simulink model "gm_Encoder_Zynq_vnl"  (R2018a)
settings: Solver=ode3  StartTime=0.0  StopTime=SimulationsDauer  RelTol=1e-3  EnableMultiTasking=on
undefined symbols (not defined in the file or in its folder): DiscIntNeverNeededParam, f_ISR, IncPerTurn, n_max, OverSamplingFactor, OverSamplingFactorInverse, Periode, Phase_Delay_A, Phase_Delay_B, PolePair, T_mech, TestDrehzahl_rpm
libraries: simulink x18, hdlsllib x2, dspsigops x2, dspswit3 x2, powerlib_meascontrol x2, hdlmdlgenlib x1, simulink_extras x1, powerlib x1
(part 2 of 3)

== system gm_Encoder_Zynq_vnl/Compare/Assert_edge ==
  cosim : Inport
  dut : Inport  Port=2
  AssertEq : Assertion  StopWhenAssertionFail=off
  Compare To Zero : simulink/Logic and Bit Operations/Compare To Zero  relop===  OutDataTypeStr=boolean
  Constant1 : Constant  Value=0  OutDataTypeStr=Inherit: Inherit via back propagation  SampleTime=-1
  Counter : simulink/Sources/Counter Free-Running  NumBits=32  tsamp=-1
  IgnoreCycles : Constant  Value=11  OutDataTypeStr=Inherit: Inherit via back propagation  SampleTime=-1
  Relational Operator : RelationalOperator  Operator=<  OutDataTypeStr=boolean  RndMeth=Nearest
  Relational Operator1 : RelationalOperator  Operator===  OutDataTypeStr=boolean  RndMeth=Nearest
  Switch : Switch  Criteria=u2 ~= 0
  Switch1 : Switch  Criteria=u2 ~= 0
  compare: edge : Scope  NumInputPorts=3
  wires:
  Compare To Zero/1 -> compare: edge/3
  Relational Operator1/1 -> Compare To Zero/1, AssertEq/1  "err"
  Switch1/1 -> compare: edge/1, Relational Operator1/1
  Switch/1 -> compare: edge/2, Relational Operator1/2
  Constant1/1 -> Switch/1, Switch1/1
  Relational Operator/1 -> Switch/2, Switch1/2
  cosim/1 -> Switch1/3  "cosim"
  dut/1 -> Switch/3  "dut ref"
  Counter/1 -> Relational Operator/1
  IgnoreCycles/1 -> Relational Operator/2

== system gm_Encoder_Zynq_vnl/Compare/Assert_omega ==
  cosim : Inport
  dut : Inport  Port=2
  AssertEq : Assertion  StopWhenAssertionFail=off
  Compare To Zero : simulink/Logic and Bit Operations/Compare To Zero  relop===  OutDataTypeStr=boolean
  Constant1 : Constant  Value=0  OutDataTypeStr=Inherit: Inherit via back propagation  SampleTime=-1
  Counter : simulink/Sources/Counter Free-Running  NumBits=32  tsamp=-1
  IgnoreCycles : Constant  Value=11  OutDataTypeStr=Inherit: Inherit via back propagation  SampleTime=-1
  Relational Operator : RelationalOperator  Operator=<  OutDataTypeStr=boolean  RndMeth=Nearest
  Relational Operator1 : RelationalOperator  Operator===  OutDataTypeStr=boolean  RndMeth=Nearest
  Switch : Switch  Criteria=u2 ~= 0
  Switch1 : Switch  Criteria=u2 ~= 0
  compare: omega : Scope  NumInputPorts=3
  wires:
  Compare To Zero/1 -> compare: omega/3
  Relational Operator1/1 -> Compare To Zero/1, AssertEq/1  "err"
  Switch1/1 -> compare: omega/1, Relational Operator1/1
  Switch/1 -> compare: omega/2, Relational Operator1/2
  Constant1/1 -> Switch/1, Switch1/1
  Relational Operator/1 -> Switch/2, Switch1/2
  cosim/1 -> Switch1/3  "cosim"
  dut/1 -> Switch/3  "dut ref"
  Counter/1 -> Relational Operator/1
  IgnoreCycles/1 -> Relational Operator/2

== system gm_Encoder_Zynq_vnl/Compare/Assert_omega_AXI4 ==
  cosim : Inport
  dut : Inport  Port=2
  AssertEq : Assertion  StopWhenAssertionFail=off
  Compare To Zero : simulink/Logic and Bit Operations/Compare To Zero  relop===  OutDataTypeStr=boolean
  Constant1 : Constant  Value=0  OutDataTypeStr=Inherit: Inherit via back propagation  SampleTime=-1
  Counter : simulink/Sources/Counter Free-Running  NumBits=32  tsamp=-1
  IgnoreCycles : Constant  Value=11  OutDataTypeStr=Inherit: Inherit via back propagation  SampleTime=-1
  Relational Operator : RelationalOperator  Operator=<  OutDataTypeStr=boolean  RndMeth=Nearest
  Relational Operator1 : RelationalOperator  Operator===  OutDataTypeStr=boolean  RndMeth=Nearest
  Switch : Switch  Criteria=u2 ~= 0
  Switch1 : Switch  Criteria=u2 ~= 0
  compare: omega_AXI4 : Scope  NumInputPorts=3
  wires:
  Compare To Zero/1 -> compare: omega_AXI4/3
  Relational Operator1/1 -> Compare To Zero/1, AssertEq/1  "err"
  Switch1/1 -> compare: omega_AXI4/1, Relational Operator1/1
  Switch/1 -> compare: omega_AXI4/2, Relational Operator1/2
  Constant1/1 -> Switch/1, Switch1/1
  Relational Operator/1 -> Switch/2, Switch1/2
  cosim/1 -> Switch1/3  "cosim"
  dut/1 -> Switch/3  "dut ref"
  Counter/1 -> Relational Operator/1
  IgnoreCycles/1 -> Relational Operator/2

== system gm_Encoder_Zynq_vnl/Compare/Assert_theta_el ==
  cosim : Inport
  dut : Inport  Port=2
  AssertEq : Assertion  StopWhenAssertionFail=off
  Compare To Zero : simulink/Logic and Bit Operations/Compare To Zero  relop===  OutDataTypeStr=boolean
  Constant1 : Constant  Value=0  OutDataTypeStr=Inherit: Inherit via back propagation  SampleTime=-1
  Counter : simulink/Sources/Counter Free-Running  NumBits=32  tsamp=-1
  IgnoreCycles : Constant  Value=11  OutDataTypeStr=Inherit: Inherit via back propagation  SampleTime=-1
  Relational Operator : RelationalOperator  Operator=<  OutDataTypeStr=boolean  RndMeth=Nearest
  Relational Operator1 : RelationalOperator  Operator===  OutDataTypeStr=boolean  RndMeth=Nearest
  Switch : Switch  Criteria=u2 ~= 0
  Switch1 : Switch  Criteria=u2 ~= 0
  compare: theta_el : Scope  NumInputPorts=3
  wires:
  Compare To Zero/1 -> compare: theta_el/3
  Relational Operator1/1 -> Compare To Zero/1, AssertEq/1  "err"
  Switch1/1 -> compare: theta_el/1, Relational Operator1/1
  Switch/1 -> compare: theta_el/2, Relational Operator1/2
  Constant1/1 -> Switch/1, Switch1/1
  Relational Operator/1 -> Switch/2, Switch1/2
  cosim/1 -> Switch1/3  "cosim"
  dut/1 -> Switch/3  "dut ref"
  Counter/1 -> Relational Operator/1
  IgnoreCycles/1 -> Relational Operator/2

== system gm_Encoder_Zynq_vnl/Compare/Assert_theta_el_AXI4 ==
  cosim : Inport
  dut : Inport  Port=2
  AssertEq : Assertion  StopWhenAssertionFail=off
  Compare To Zero : simulink/Logic and Bit Operations/Compare To Zero  relop===  OutDataTypeStr=boolean
  Constant1 : Constant  Value=0  OutDataTypeStr=Inherit: Inherit via back propagation  SampleTime=-1
  Counter : simulink/Sources/Counter Free-Running  NumBits=32  tsamp=-1
  IgnoreCycles : Constant  Value=11  OutDataTypeStr=Inherit: Inherit via back propagation  SampleTime=-1
  Relational Operator : RelationalOperator  Operator=<  OutDataTypeStr=boolean  RndMeth=Nearest
  Relational Operator1 : RelationalOperator  Operator===  OutDataTypeStr=boolean  RndMeth=Nearest
  Switch : Switch  Criteria=u2 ~= 0
  Switch1 : Switch  Criteria=u2 ~= 0
  compare: theta_el_AXI4 : Scope  NumInputPorts=3
  wires:
  Compare To Zero/1 -> compare: theta_el_AXI4/3
  Relational Operator1/1 -> Compare To Zero/1, AssertEq/1  "err"
  Switch1/1 -> compare: theta_el_AXI4/1, Relational Operator1/1
  Switch/1 -> compare: theta_el_AXI4/2, Relational Operator1/2
  Constant1/1 -> Switch/1, Switch1/1
  Relational Operator/1 -> Switch/2, Switch1/2
  cosim/1 -> Switch1/3  "cosim"
  dut/1 -> Switch/3  "dut ref"
  Counter/1 -> Relational Operator/1
  IgnoreCycles/1 -> Relational Operator/2

== system gm_Encoder_Zynq_vnl/Compare/Assert_theta_mech_AXI4 ==
  cosim : Inport
  dut : Inport  Port=2
  AssertEq : Assertion  StopWhenAssertionFail=off
  Compare To Zero : simulink/Logic and Bit Operations/Compare To Zero  relop===  OutDataTypeStr=boolean
  Constant1 : Constant  Value=0  OutDataTypeStr=Inherit: Inherit via back propagation  SampleTime=-1
  Counter : simulink/Sources/Counter Free-Running  NumBits=32  tsamp=-1
  IgnoreCycles : Constant  Value=11  OutDataTypeStr=Inherit: Inherit via back propagation  SampleTime=-1
  Relational Operator : RelationalOperator  Operator=<  OutDataTypeStr=boolean  RndMeth=Nearest
  Relational Operator1 : RelationalOperator  Operator===  OutDataTypeStr=boolean  RndMeth=Nearest
  Switch : Switch  Criteria=u2 ~= 0
  Switch1 : Switch  Criteria=u2 ~= 0
  compare: theta_mech_AXI4 : Scope  NumInputPorts=3
  wires:
  Compare To Zero/1 -> compare: theta_mech_AXI4/3
  Relational Operator1/1 -> Compare To Zero/1, AssertEq/1  "err"
  Switch1/1 -> compare: theta_mech_AXI4/1, Relational Operator1/1
  Switch/1 -> compare: theta_mech_AXI4/2, Relational Operator1/2
  Constant1/1 -> Switch/1, Switch1/1
  Relational Operator/1 -> Switch/2, Switch1/2
  cosim/1 -> Switch1/3  "cosim"
  dut/1 -> Switch/3  "dut ref"
  Counter/1 -> Relational Operator/1
  IgnoreCycles/1 -> Relational Operator/2

== system gm_Encoder_Zynq_vnl/Compare/CleanupScopes ==

== system gm_Encoder_Zynq_vnl/Compare/Enable ==

== system gm_Encoder_Zynq_vnl/IncreEncoder_V16/Check_Direction ==
  A : Inport
  B : Inport  Port=2
  Add : Sum  Inputs=+-  AccumDataTypeStr=fixdt(1,4,0)  OutDataTypeStr=fixdt(1,4,0)
  Add1 : Sum  Inputs=+-  AccumDataTypeStr=fixdt(1,4,0)  OutDataTypeStr=fixdt(1,4,0)
  Add2 : Sum  AccumDataTypeStr=fixdt(1,4,0)  OutDataTypeStr=fixdt(1,4,0)
  Change : Sum  AccumDataTypeStr=fixdt(1,4,0)  OutDataTypeStr=fixdt(1,4,0)
  Change1 : Delay  DelayLength=1
  Save_Direction : Switch  Criteria=u2 ~= 0  Threshold=0.1  OutDataTypeStr=Inherit: Inherit via back propagation
  Scope6 : Scope  NumInputPorts=4
  T_count_switch : Switch  Threshold=1  OutDataTypeStr=Inherit: Inherit via back propagation
  TrnLeft : Sum  Inputs=+-  AccumDataTypeStr=fixdt(1,4,0)  OutDataTypeStr=fixdt(1,4,0)
  TrnRight : Sum  Inputs=+-  AccumDataTypeStr=fixdt(1,4,0)  OutDataTypeStr=fixdt(1,4,0)
  TurnLeft : Constant  Value=-1  OutDataTypeStr=fixdt(1,4,0)  SampleTime=-1
  TurnRight : Constant  OutDataTypeStr=fixdt(1,4,0)  SampleTime=-1
  count_old : Delay  DelayLength=1
  count_old1 : Delay  DelayLength=1
  count_old2 : Delay  DelayLength=1
  count_old_switch : Switch  Criteria=u2 ~= 0  OutDataTypeStr=Inherit: Inherit via back propagation
  count_old_switch1 : Switch  Criteria=u2 ~= 0  OutDataTypeStr=Inherit: Inherit via back propagation
  new_value : Delay  DelayLength=1
  nothing : Constant  Value=0  OutDataTypeStr=fixdt(1,4,0)  SampleTime=-1
  nothing1 : Constant  Value=0  OutDataTypeStr=fixdt(1,4,0)  SampleTime=-1
  speed_old_switch : Switch  Threshold=1  OutDataTypeStr=Inherit: Inherit via back propagation
  Dir : Outport
  wires:
  A/1 -> TrnLeft/2, Add/1, count_old_switch/1
  count_old_switch/1 -> count_old/1
  count_old/1 -> count_old_switch/3, Add/2
  TurnRight/1 -> T_count_switch/1
  Add/1 -> TrnRight/1, count_old_switch/2
  T_count_switch/1 -> Change/1, Add2/1
  Save_Direction/1 -> count_old2/1
  B/1 -> TrnRight/2, Add1/1, count_old_switch1/1
  count_old_switch1/1 -> count_old1/1
  count_old1/1 -> count_old_switch1/3, Add1/2
  Add1/1 -> TrnLeft/1, count_old_switch1/2
  TrnRight/1 -> Scope6/1, T_count_switch/2
  new_value/1 -> Save_Direction/1
  TrnLeft/1 -> speed_old_switch/2, Scope6/2
  TurnLeft/1 -> speed_old_switch/1
  nothing/1 -> speed_old_switch/3
  nothing1/1 -> T_count_switch/3
  speed_old_switch/1 -> Change/2, Add2/2
  Add2/1 -> Scope6/4, new_value/1
  Change/1 -> Change1/1
  Change1/1 -> Scope6/3, Save_Direction/2
  count_old2/1 -> Save_Direction/3, Dir/1

== system gm_Encoder_Zynq_vnl/IncreEncoder_V16/Counter_speed ==
  note: 1 for one cycle if edge recognized
  note: Check if count is to small
  note: Check if count is to big
  note: Reset
  note: Count
  Enable_ctr : Inport
  Reset : Inport  Port=2
  IncsPerTurn : Inport  Port=3
  Add1 : Sum  AccumDataTypeStr=int16  OutDataTypeStr=uint16
  Constant1 : Constant  Value=0  OutDataTypeStr=uint16  SampleTime=-1
  Constant2 : Constant  OutDataTypeStr=int8  SampleTime=-1
  Constant3 : Constant  Value=0  OutDataTypeStr=int8  SampleTime=-1
  Constant4 : Constant  Value=10  OutDataTypeStr=uint16  SampleTime=-1
  Detec_edge : Sum  Inputs=+-  AccumDataTypeStr=int8  OutDataTypeStr=int8
  Relational Operator : RelationalOperator  OutDataTypeStr=boolean  RndMeth=Nearest
  Reset_flag : Sum  Inputs=+-  AccumDataTypeStr=uint8  OutDataTypeStr=uint8
  Reset_when_overflow : Sum
  Resett_switch1 : Switch  Criteria=u2 ~= 0
  Resett_switch2 : Switch  Criteria=u2 ~= 0
  reset_old{,1..3} (4 alike) : Delay  DelayLength=1
  reset_old_switch : Switch  Criteria=u2 ~= 0
  reset_old_switch1 : Switch  Criteria=u2 ~= 0
  speed_old_switch1 : Switch  Threshold=1
  count : Outport
  wires:
  Reset/1 -> Reset_flag/1, reset_old_switch/1
  reset_old_switch/1 -> reset_old/1
  reset_old/1 -> reset_old_switch/3, Reset_flag/2
  Reset_flag/1 -> reset_old_switch/2, Resett_switch2/2
  Enable_ctr/1 -> Detec_edge/1, reset_old_switch1/1
  reset_old_switch1/1 -> reset_old1/1
  reset_old1/1 -> reset_old_switch1/3, Detec_edge/2
  Detec_edge/1 -> speed_old_switch1/2, reset_old_switch1/2  "1 for one cycle if edge recognized"
  Add1/1 -> Resett_switch2/3
  reset_old2/1 -> Relational Operator/1, Add1/2, count/1
  speed_old_switch1/1 -> Add1/1
  Constant3/1 -> speed_old_switch1/3
  Constant2/1 -> speed_old_switch1/1
  Constant4/1 -> Reset_when_overflow/1
  Reset_when_overflow/1 -> reset_old3/1
  Resett_switch1/1 -> reset_old2/1
  Relational Operator/1 -> Resett_switch1/2
  Constant1/1 -> Resett_switch2/1, Resett_switch1/1
  IncsPerTurn/1 -> Reset_when_overflow/2
  Resett_switch2/1 -> Resett_switch1/3
  reset_old3/1 -> Relational Operator/2

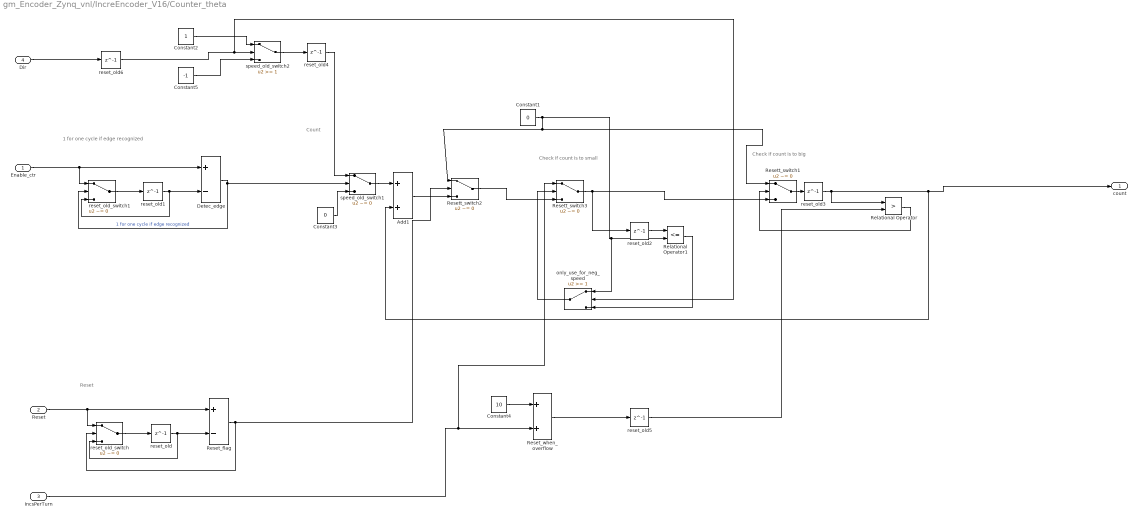
== system gm_Encoder_Zynq_vnl/IncreEncoder_V16/Counter_theta ==
  note: 1 for one cycle if edge recognized
  note: Reset
  note: Count
  note: Check if count is to big
  note: Check if count is to small
  Enable_ctr : Inport
  Reset : Inport  Port=2
  IncsPerTurn : Inport  Port=3
  Dir : Inport  Port=4
  Add1 : Sum  AccumDataTypeStr=int16  OutDataTypeStr=int16
  Constant1 : Constant  Value=0  OutDataTypeStr=int16  SampleTime=-1
  Constant2 : Constant  OutDataTypeStr=int16  SampleTime=-1
  Constant3 : Constant  Value=0  OutDataTypeStr=int16  SampleTime=-1
  Constant4 : Constant  Value=10  OutDataTypeStr=int16  SampleTime=-1
  Constant5 : Constant  Value=-1  OutDataTypeStr=int16  SampleTime=-1
  Detec_edge : Sum  Inputs=+-  AccumDataTypeStr=int8  OutDataTypeStr=int8
  Relational Operator : RelationalOperator  Operator=>  OutDataTypeStr=boolean  RndMeth=Nearest
  Relational Operator1 : RelationalOperator  Operator=<=  OutDataTypeStr=boolean  RndMeth=Nearest
  Reset_flag : Sum  Inputs=+-  AccumDataTypeStr=uint8  OutDataTypeStr=uint8
  Reset_when_overflow : Sum  OutDataTypeStr=int16
  Resett_switch1 : Switch  Criteria=u2 ~= 0  OutDataTypeStr=int16
  Resett_switch2 : Switch  Criteria=u2 ~= 0  OutDataTypeStr=int16
  Resett_switch3 : Switch  Criteria=u2 ~= 0  OutDataTypeStr=int16
  only_use_for_neg_speed : Switch  Threshold=1
  reset_old{,1..6} (7 alike) : Delay  DelayLength=1
  reset_old_switch : Switch  Criteria=u2 ~= 0
  reset_old_switch1 : Switch  Criteria=u2 ~= 0
  speed_old_switch1 : Switch  Criteria=u2 ~= 0
  speed_old_switch2 : Switch  Threshold=1
  count : Outport
  wires:
  Reset/1 -> Reset_flag/1, reset_old_switch/1
  reset_old_switch/1 -> reset_old/1
  reset_old/1 -> reset_old_switch/3, Reset_flag/2
  Reset_flag/1 -> reset_old_switch/2, Resett_switch2/2
  Enable_ctr/1 -> Detec_edge/1, reset_old_switch1/1
  reset_old_switch1/1 -> reset_old1/1
  reset_old1/1 -> reset_old_switch1/3, Detec_edge/2
  Detec_edge/1 -> speed_old_switch1/2, reset_old_switch1/2  "1 for one cycle if edge recognized"
  Add1/1 -> Resett_switch2/3
  speed_old_switch1/1 -> Add1/1
  Constant3/1 -> speed_old_switch1/3
  Constant2/1 -> speed_old_switch2/1
  Constant4/1 -> Reset_when_overflow/1
  Reset_when_overflow/1 -> reset_old5/1
  IncsPerTurn/1 -> Resett_switch3/1, Reset_when_overflow/2
  Dir/1 -> reset_old6/1
  Constant5/1 -> speed_old_switch2/3
  speed_old_switch2/1 -> reset_old4/1
  reset_old3/1 -> Add1/2, count/1, Relational Operator/1
  Resett_switch1/1 -> reset_old3/1
  Relational Operator/1 -> Resett_switch1/2
  Constant1/1 -> Resett_switch2/1, Resett_switch1/1, only_use_for_neg_speed/1, Relational Operator1/2
  Resett_switch3/1 -> reset_old2/1, Resett_switch1/3
  Resett_switch2/1 -> Resett_switch3/3
  reset_old2/1 -> Relational Operator1/1
  Relational Operator1/1 -> only_use_for_neg_speed/3
  only_use_for_neg_speed/1 -> Resett_switch3/2
  reset_old4/1 -> speed_old_switch1/1
  reset_old5/1 -> Relational Operator/2
  reset_old6/1 -> only_use_for_neg_speed/2, speed_old_switch2/2

== system gm_Encoder_Zynq_vnl/IncreEncoder_V16/Counter_theta_ele ==
  note: 1 for one cycle if edge recognized
  note: Reset
  note: Count
  note: Check if count is to big
  note: Check if count is to small
  Enable_ctr : Inport
  Reset : Inport  Port=2
  IncsPerTurn : Inport  Port=3
  Dir : Inport  Port=4
  Add1 : Sum  AccumDataTypeStr=int16  OutDataTypeStr=int16
  Constant1 : Constant  Value=0  OutDataTypeStr=int16  SampleTime=-1
  Constant2 : Constant  OutDataTypeStr=int16  SampleTime=-1
  Constant3 : Constant  Value=0  OutDataTypeStr=int16  SampleTime=-1
  Constant5 : Constant  Value=-1  OutDataTypeStr=int16  SampleTime=-1
  Detec_edge : Sum  Inputs=+-  AccumDataTypeStr=int8  OutDataTypeStr=int8
  Relational Operator : RelationalOperator  Operator=>  OutDataTypeStr=boolean  RndMeth=Nearest
  Relational Operator1 : RelationalOperator  Operator=<=  OutDataTypeStr=boolean  RndMeth=Nearest
  Reset_flag : Sum  Inputs=+-  AccumDataTypeStr=uint8  OutDataTypeStr=uint8
  Resett_switch1 : Switch  Criteria=u2 ~= 0  OutDataTypeStr=int16
  Resett_switch2 : Switch  Criteria=u2 ~= 0  OutDataTypeStr=int16
  Resett_switch3 : Switch  Criteria=u2 ~= 0  OutDataTypeStr=int16
  only_use_for_neg_speed : Switch  Threshold=1
  reset_old{,1..5} (6 alike) : Delay  DelayLength=1
  reset_old_switch : Switch  Criteria=u2 ~= 0
  reset_old_switch1 : Switch  Criteria=u2 ~= 0
  speed_old_switch1 : Switch  Criteria=u2 ~= 0
  speed_old_switch2 : Switch  Threshold=1
  count : Outport
  wires:
  Reset/1 -> Reset_flag/1, reset_old_switch/1
  reset_old_switch/1 -> reset_old/1
  reset_old/1 -> reset_old_switch/3, Reset_flag/2
  Reset_flag/1 -> reset_old_switch/2, Resett_switch2/2
  Enable_ctr/1 -> Detec_edge/1, reset_old_switch1/1
  reset_old_switch1/1 -> reset_old1/1
  reset_old1/1 -> reset_old_switch1/3, Detec_edge/2
  Detec_edge/1 -> speed_old_switch1/2, reset_old_switch1/2  "1 for one cycle if edge recognized"
  Add1/1 -> Resett_switch2/3
  speed_old_switch1/1 -> Add1/1
  Constant3/1 -> speed_old_switch1/3
  Constant2/1 -> speed_old_switch2/1
  IncsPerTurn/1 -> Resett_switch3/1, Relational Operator/2
  Dir/1 -> reset_old5/1
  Constant5/1 -> speed_old_switch2/3
  speed_old_switch2/1 -> reset_old4/1
  reset_old3/1 -> Add1/2, count/1, Relational Operator/1
  Resett_switch1/1 -> reset_old3/1
  Relational Operator/1 -> Resett_switch1/2
  Constant1/1 -> Resett_switch2/1, only_use_for_neg_speed/1, Relational Operator1/2, Resett_switch1/1
  Resett_switch3/1 -> reset_old2/1, Resett_switch1/3
  Resett_switch2/1 -> Resett_switch3/3
  reset_old2/1 -> Relational Operator1/1
  Relational Operator1/1 -> only_use_for_neg_speed/3
  only_use_for_neg_speed/1 -> Resett_switch3/2
  reset_old4/1 -> speed_old_switch1/1
  reset_old5/1 -> speed_old_switch2/2, only_use_for_neg_speed/2

== system gm_Encoder_Zynq_vnl/IncreEncoder_V16/n_aus_theta ==
  count : Inport
  IncsPerTurn : Inport  Port=2
  T : Inport  Port=3
  Add : Sum  Inputs=+-
  Add1 : Sum
  Constant : Constant  Value=0  OutDataTypeStr=fixdt(0,30,24)  SampleTime=-1
  Constant1 : Constant  Value=0  OutDataTypeStr=fixdt(0,30,24)  SampleTime=-1
  Constant2 : Constant  Value=0  OutDataTypeStr=fixdt(0,30,24)  SampleTime=-1
  Gain : Gain  Gain=0.001  ParamDataTypeStr=fixdt(0,16)  OutMin=0  OutMax=0.001*2^16  OutDataTypeStr=fixdt(0,18)
  Product : Product  OutDataTypeStr=Inherit: Same as first input
  ProtectOverflow_T_count : Switch  Threshold=50
  ProtectOverflow_rps : Switch  Threshold=50  OutDataTypeStr=fixdt(0,30,24)
  T_count : Delay  DelayLength=1
  T_count_switch : Switch  Criteria=u2 ~= 0
  count_old : Delay  DelayLength=1
  count_old_switch : Switch  Criteria=u2 ~= 0
  speed_old : Delay  DelayLength=1
  speed_old_switch : Switch  Criteria=u2 ~= 0
  rps : Outport
  wires:
  count_old_switch/1 -> count_old/1
  count_old/1 -> count_old_switch/3, Add/2
  Constant/1 -> T_count_switch/1
  Add/1 -> speed_old_switch/2, count_old_switch/2, T_count_switch/2
  Constant1/1 -> ProtectOverflow_T_count/1
  ProtectOverflow_rps/1 -> rps/1
  Constant2/1 -> ProtectOverflow_rps/1
  speed_old_switch/1 -> ProtectOverflow_rps/3, speed_old/1
  speed_old/1 -> speed_old_switch/3
  IncsPerTurn/1 -> Gain/1
  Gain/1 -> Product/2
  T/1 -> Add1/1
  ProtectOverflow_T_count/1 -> T_count/1
  T_count/1 -> Add1/2
  Product/1 -> speed_old_switch/1
  Add1/1 -> Product/1, T_count_switch/3
  count/1 -> Add/1, count_old_switch/1
  T_count_switch/1 -> ProtectOverflow_rps/2, ProtectOverflow_T_count/2, ProtectOverflow_T_count/3

== system gm_Encoder_Zynq_vnl/IncreEncoder_V18/Check_Direction ==
  A : Inport
  B : Inport  Port=2
  Add : Sum  Inputs=+-  AccumDataTypeStr=fixdt(1,4,0)  OutDataTypeStr=fixdt(1,4,0)
  Add1 : Sum  Inputs=+-  AccumDataTypeStr=fixdt(1,4,0)  OutDataTypeStr=fixdt(1,4,0)
  Add2 : Sum  AccumDataTypeStr=fixdt(1,4,0)  OutDataTypeStr=fixdt(1,4,0)
  Change : Sum  AccumDataTypeStr=fixdt(1,4,0)  OutDataTypeStr=fixdt(1,4,0)
  Change1 : Delay  DelayLength=1
  Save_Direction : Switch  Criteria=u2 ~= 0  Threshold=0.1  OutDataTypeStr=Inherit: Inherit via back propagation
  Scope6 : Scope  NumInputPorts=4
  T_count_switch : Switch  Threshold=1  OutDataTypeStr=Inherit: Inherit via back propagation
  TrnLeft : Sum  Inputs=+-  AccumDataTypeStr=fixdt(1,4,0)  OutDataTypeStr=fixdt(1,4,0)
  TrnRight : Sum  Inputs=+-  AccumDataTypeStr=fixdt(1,4,0)  OutDataTypeStr=fixdt(1,4,0)
  TurnLeft : Constant  Value=-1  OutDataTypeStr=fixdt(1,4,0)  SampleTime=-1
  TurnRight : Constant  OutDataTypeStr=fixdt(1,4,0)  SampleTime=-1
  count_old : Delay  DelayLength=1
  count_old1 : Delay  DelayLength=1
  count_old2 : Delay  DelayLength=1
  count_old_switch : Switch  Criteria=u2 ~= 0  OutDataTypeStr=Inherit: Inherit via back propagation
  count_old_switch1 : Switch  Criteria=u2 ~= 0  OutDataTypeStr=Inherit: Inherit via back propagation
  new_value : Delay  DelayLength=1
  nothing : Constant  Value=0  OutDataTypeStr=fixdt(1,4,0)  SampleTime=-1
  nothing1 : Constant  Value=0  OutDataTypeStr=fixdt(1,4,0)  SampleTime=-1
  speed_old_switch : Switch  Threshold=1  OutDataTypeStr=Inherit: Inherit via back propagation
  Dir : Outport
  wires:
  A/1 -> TrnLeft/2, Add/1, count_old_switch/1
  count_old_switch/1 -> count_old/1
  count_old/1 -> count_old_switch/3, Add/2
  TurnRight/1 -> T_count_switch/1
  Add/1 -> TrnRight/1, count_old_switch/2
  T_count_switch/1 -> Change/1, Add2/1
  Save_Direction/1 -> count_old2/1
  B/1 -> TrnRight/2, Add1/1, count_old_switch1/1
  count_old_switch1/1 -> count_old1/1
  count_old1/1 -> count_old_switch1/3, Add1/2
  Add1/1 -> TrnLeft/1, count_old_switch1/2
  TrnRight/1 -> Scope6/1, T_count_switch/2
  new_value/1 -> Save_Direction/1
  TrnLeft/1 -> speed_old_switch/2, Scope6/2
  TurnLeft/1 -> speed_old_switch/1
  nothing/1 -> speed_old_switch/3
  nothing1/1 -> T_count_switch/3
  speed_old_switch/1 -> Change/2, Add2/2
  Add2/1 -> Scope6/4, new_value/1
  Change/1 -> Change1/1
  Change1/1 -> Scope6/3, Save_Direction/2
  count_old2/1 -> Save_Direction/3, Dir/1

== system gm_Encoder_Zynq_vnl/IncreEncoder_V18/Counter_speed ==
  note: 1 for one cycle if edge recognized
  note: Check if count is to small
  note: Check if count is to big
  note: Reset
  note: Count
  Enable_ctr : Inport
  Reset : Inport  Port=2
  IncsPerTurn : Inport  Port=3
  Add1 : Sum  AccumDataTypeStr=int16  OutDataTypeStr=uint16
  Constant1 : Constant  Value=0  OutDataTypeStr=uint16  SampleTime=-1
  Constant2 : Constant  OutDataTypeStr=int8  SampleTime=-1
  Constant3 : Constant  Value=0  OutDataTypeStr=int8  SampleTime=-1
  Constant4 : Constant  Value=10  OutDataTypeStr=uint16  SampleTime=-1
  Detec_edge : Sum  Inputs=+-  AccumDataTypeStr=int8  OutDataTypeStr=int8
  Relational Operator : RelationalOperator  OutDataTypeStr=boolean  RndMeth=Nearest
  Reset_flag : Sum  Inputs=+-  AccumDataTypeStr=uint8  OutDataTypeStr=uint8
  Reset_when_overflow : Sum
  Resett_switch1 : Switch  Criteria=u2 ~= 0
  Resett_switch2 : Switch  Criteria=u2 ~= 0
  reset_old{,1..3} (4 alike) : Delay  DelayLength=1
  reset_old_switch : Switch  Criteria=u2 ~= 0
  reset_old_switch1 : Switch  Criteria=u2 ~= 0
  speed_old_switch1 : Switch  Threshold=1
  count : Outport
  wires:
  Reset/1 -> Reset_flag/1, reset_old_switch/1
  reset_old_switch/1 -> reset_old/1
  reset_old/1 -> reset_old_switch/3, Reset_flag/2
  Reset_flag/1 -> reset_old_switch/2, Resett_switch2/2
  Enable_ctr/1 -> Detec_edge/1, reset_old_switch1/1
  reset_old_switch1/1 -> reset_old1/1
  reset_old1/1 -> reset_old_switch1/3, Detec_edge/2
  Detec_edge/1 -> speed_old_switch1/2, reset_old_switch1/2  "1 for one cycle if edge recognized"
  Add1/1 -> Resett_switch2/3
  reset_old2/1 -> Relational Operator/1, Add1/2, count/1
  speed_old_switch1/1 -> Add1/1
  Constant3/1 -> speed_old_switch1/3
  Constant2/1 -> speed_old_switch1/1
  Constant4/1 -> Reset_when_overflow/1
  Reset_when_overflow/1 -> reset_old3/1
  Resett_switch1/1 -> reset_old2/1
  Relational Operator/1 -> Resett_switch1/2
  Constant1/1 -> Resett_switch2/1, Resett_switch1/1
  IncsPerTurn/1 -> Reset_when_overflow/2
  Resett_switch2/1 -> Resett_switch1/3
  reset_old3/1 -> Relational Operator/2

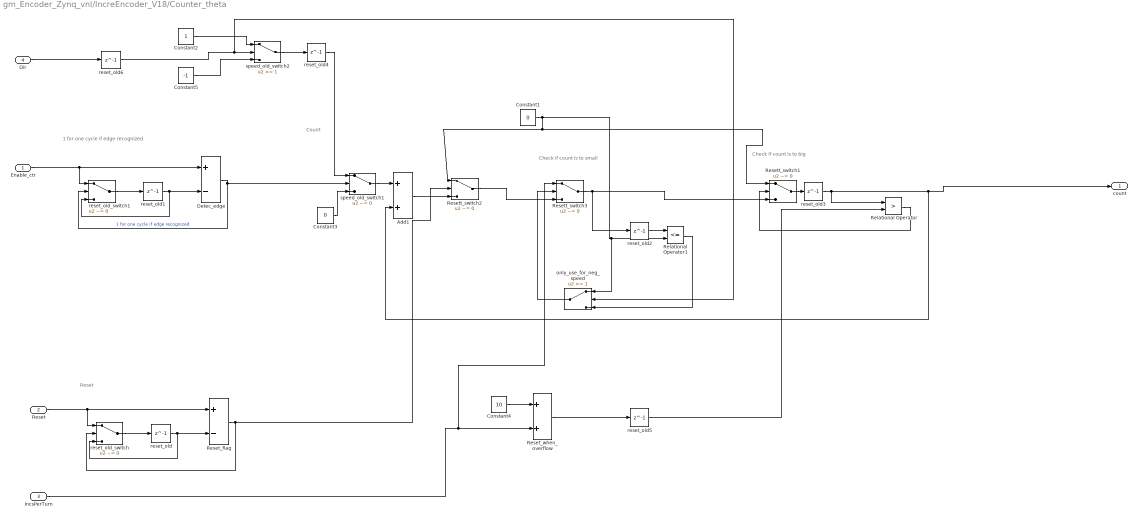
== system gm_Encoder_Zynq_vnl/IncreEncoder_V18/Counter_theta ==
  note: 1 for one cycle if edge recognized
  note: Reset
  note: Count
  note: Check if count is to big
  note: Check if count is to small
  Enable_ctr : Inport
  Reset : Inport  Port=2
  IncsPerTurn : Inport  Port=3
  Dir : Inport  Port=4
  Add1 : Sum  AccumDataTypeStr=int16  OutDataTypeStr=int16
  Constant1 : Constant  Value=0  OutDataTypeStr=int16  SampleTime=-1
  Constant2 : Constant  OutDataTypeStr=int16  SampleTime=-1
  Constant3 : Constant  Value=0  OutDataTypeStr=int16  SampleTime=-1
  Constant4 : Constant  Value=10  OutDataTypeStr=int16  SampleTime=-1
  Constant5 : Constant  Value=-1  OutDataTypeStr=int16  SampleTime=-1
  Detec_edge : Sum  Inputs=+-  AccumDataTypeStr=int8  OutDataTypeStr=int8
  Relational Operator : RelationalOperator  Operator=>  OutDataTypeStr=boolean  RndMeth=Nearest
  Relational Operator1 : RelationalOperator  Operator=<=  OutDataTypeStr=boolean  RndMeth=Nearest
  Reset_flag : Sum  Inputs=+-  AccumDataTypeStr=uint8  OutDataTypeStr=uint8
  Reset_when_overflow : Sum  OutDataTypeStr=int16
  Resett_switch1 : Switch  Criteria=u2 ~= 0  OutDataTypeStr=int16
  Resett_switch2 : Switch  Criteria=u2 ~= 0  OutDataTypeStr=int16
  Resett_switch3 : Switch  Criteria=u2 ~= 0  OutDataTypeStr=int16
  only_use_for_neg_speed : Switch  Threshold=1
  reset_old{,1..6} (7 alike) : Delay  DelayLength=1
  reset_old_switch : Switch  Criteria=u2 ~= 0
  reset_old_switch1 : Switch  Criteria=u2 ~= 0
  speed_old_switch1 : Switch  Criteria=u2 ~= 0
  speed_old_switch2 : Switch  Threshold=1
  count : Outport
  wires:
  Reset/1 -> Reset_flag/1, reset_old_switch/1
  reset_old_switch/1 -> reset_old/1
  reset_old/1 -> reset_old_switch/3, Reset_flag/2
  Reset_flag/1 -> reset_old_switch/2, Resett_switch2/2
  Enable_ctr/1 -> Detec_edge/1, reset_old_switch1/1
  reset_old_switch1/1 -> reset_old1/1
  reset_old1/1 -> reset_old_switch1/3, Detec_edge/2
  Detec_edge/1 -> speed_old_switch1/2, reset_old_switch1/2  "1 for one cycle if edge recognized"
  Add1/1 -> Resett_switch2/3
  speed_old_switch1/1 -> Add1/1
  Constant3/1 -> speed_old_switch1/3
  Constant2/1 -> speed_old_switch2/1
  Constant4/1 -> Reset_when_overflow/1
  Reset_when_overflow/1 -> reset_old5/1
  IncsPerTurn/1 -> Resett_switch3/1, Reset_when_overflow/2
  Dir/1 -> reset_old6/1
  Constant5/1 -> speed_old_switch2/3
  speed_old_switch2/1 -> reset_old4/1
  reset_old3/1 -> Add1/2, count/1, Relational Operator/1
  Resett_switch1/1 -> reset_old3/1
  Relational Operator/1 -> Resett_switch1/2
  Constant1/1 -> Resett_switch2/1, Resett_switch1/1, only_use_for_neg_speed/1, Relational Operator1/2
  Resett_switch3/1 -> reset_old2/1, Resett_switch1/3
  Resett_switch2/1 -> Resett_switch3/3
  reset_old2/1 -> Relational Operator1/1
  Relational Operator1/1 -> only_use_for_neg_speed/3
  only_use_for_neg_speed/1 -> Resett_switch3/2
  reset_old4/1 -> speed_old_switch1/1
  reset_old5/1 -> Relational Operator/2
  reset_old6/1 -> only_use_for_neg_speed/2, speed_old_switch2/2

== system gm_Encoder_Zynq_vnl/IncreEncoder_V18/Counter_theta_ele ==
  note: 1 for one cycle if edge recognized
  note: Reset
  note: Count
  note: Check if count is to big
  note: Check if count is to small
  Enable_ctr : Inport
  Reset : Inport  Port=2
  IncsPerTurn : Inport  Port=3
  Dir : Inport  Port=4
  Add1 : Sum  AccumDataTypeStr=int16  OutDataTypeStr=int16
  Constant1 : Constant  Value=0  OutDataTypeStr=int16  SampleTime=-1
  Constant2 : Constant  OutDataTypeStr=int16  SampleTime=-1
  Constant3 : Constant  Value=0  OutDataTypeStr=int16  SampleTime=-1
  Constant5 : Constant  Value=-1  OutDataTypeStr=int16  SampleTime=-1
  Detec_edge : Sum  Inputs=+-  AccumDataTypeStr=int8  OutDataTypeStr=int8
  Relational Operator : RelationalOperator  Operator=>  OutDataTypeStr=boolean  RndMeth=Nearest
  Relational Operator1 : RelationalOperator  Operator=<=  OutDataTypeStr=boolean  RndMeth=Nearest
  Reset_flag : Sum  Inputs=+-  AccumDataTypeStr=uint8  OutDataTypeStr=uint8
  Resett_switch1 : Switch  Criteria=u2 ~= 0  OutDataTypeStr=int16
  Resett_switch2 : Switch  Criteria=u2 ~= 0  OutDataTypeStr=int16
  Resett_switch3 : Switch  Criteria=u2 ~= 0  OutDataTypeStr=int16
  only_use_for_neg_speed : Switch  Threshold=1
  reset_old{,1..5} (6 alike) : Delay  DelayLength=1
  reset_old_switch : Switch  Criteria=u2 ~= 0
  reset_old_switch1 : Switch  Criteria=u2 ~= 0
  speed_old_switch1 : Switch  Criteria=u2 ~= 0
  speed_old_switch2 : Switch  Threshold=1
  count : Outport
  wires:
  Reset/1 -> Reset_flag/1, reset_old_switch/1
  reset_old_switch/1 -> reset_old/1
  reset_old/1 -> reset_old_switch/3, Reset_flag/2
  Reset_flag/1 -> reset_old_switch/2, Resett_switch2/2
  Enable_ctr/1 -> Detec_edge/1, reset_old_switch1/1
  reset_old_switch1/1 -> reset_old1/1
  reset_old1/1 -> reset_old_switch1/3, Detec_edge/2
  Detec_edge/1 -> speed_old_switch1/2, reset_old_switch1/2  "1 for one cycle if edge recognized"
  Add1/1 -> Resett_switch2/3
  speed_old_switch1/1 -> Add1/1
  Constant3/1 -> speed_old_switch1/3
  Constant2/1 -> speed_old_switch2/1
  IncsPerTurn/1 -> Resett_switch3/1, Relational Operator/2
  Dir/1 -> reset_old5/1
  Constant5/1 -> speed_old_switch2/3
  speed_old_switch2/1 -> reset_old4/1
  reset_old3/1 -> Add1/2, count/1, Relational Operator/1
  Resett_switch1/1 -> reset_old3/1
  Relational Operator/1 -> Resett_switch1/2
  Constant1/1 -> Resett_switch2/1, only_use_for_neg_speed/1, Relational Operator1/2, Resett_switch1/1
  Resett_switch3/1 -> reset_old2/1, Resett_switch1/3
  Resett_switch2/1 -> Resett_switch3/3
  reset_old2/1 -> Relational Operator1/1
  Relational Operator1/1 -> only_use_for_neg_speed/3
  only_use_for_neg_speed/1 -> Resett_switch3/2
  reset_old4/1 -> speed_old_switch1/1
  reset_old5/1 -> speed_old_switch2/2, only_use_for_neg_speed/2

== system gm_Encoder_Zynq_vnl/IncreEncoder_V18/n_aus_theta ==
  count : Inport
  IncsPerTurn : Inport  Port=2
  T : Inport  Port=3
  Add : Sum  Inputs=+-
  Add1 : Sum
  Constant : Constant  Value=0  OutDataTypeStr=fixdt(0,30,24)  SampleTime=-1
  Constant1 : Constant  Value=0  OutDataTypeStr=fixdt(0,30,24)  SampleTime=-1
  Constant2 : Constant  Value=0  OutDataTypeStr=fixdt(0,30,24)  SampleTime=-1
  Gain : Gain  Gain=0.001  ParamDataTypeStr=fixdt(0,16)  OutMin=0  OutMax=0.001*2^16  OutDataTypeStr=fixdt(0,18)
  Product : Product  OutDataTypeStr=Inherit: Same as first input
  ProtectOverflow_T_count : Switch  Threshold=50
  ProtectOverflow_rps : Switch  Threshold=50  OutDataTypeStr=fixdt(0,30,24)
  T_count : Delay  DelayLength=1
  T_count_switch : Switch  Criteria=u2 ~= 0
  count_old : Delay  DelayLength=1
  count_old_switch : Switch  Criteria=u2 ~= 0
  speed_old : Delay  DelayLength=1
  speed_old_switch : Switch  Criteria=u2 ~= 0
  rps : Outport
  wires:
  count_old_switch/1 -> count_old/1
  count_old/1 -> count_old_switch/3, Add/2
  Constant/1 -> T_count_switch/1
  Add/1 -> speed_old_switch/2, count_old_switch/2, T_count_switch/2
  Constant1/1 -> ProtectOverflow_T_count/1
  ProtectOverflow_rps/1 -> rps/1
  Constant2/1 -> ProtectOverflow_rps/1
  speed_old_switch/1 -> ProtectOverflow_rps/3, speed_old/1
  speed_old/1 -> speed_old_switch/3
  IncsPerTurn/1 -> Gain/1
  Gain/1 -> Product/2
  T/1 -> Add1/1
  ProtectOverflow_T_count/1 -> T_count/1
  T_count/1 -> Add1/2
  Product/1 -> speed_old_switch/1
  Add1/1 -> Product/1, T_count_switch/3
  count/1 -> Add/1, count_old_switch/1
  T_count_switch/1 -> ProtectOverflow_rps/2, ProtectOverflow_T_count/2, ProtectOverflow_T_count/3

== system gm_Encoder_Zynq_vnl/IncreEncoder_V19/Check_Direction ==
  A : Inport
  B : Inport  Port=2
  Add : Sum  Inputs=+-  AccumDataTypeStr=fixdt(1,4,0)  OutDataTypeStr=fixdt(1,4,0)
  Add1 : Sum  Inputs=+-  AccumDataTypeStr=fixdt(1,4,0)  OutDataTypeStr=fixdt(1,4,0)
  Add2 : Sum  AccumDataTypeStr=fixdt(1,4,0)  OutDataTypeStr=fixdt(1,4,0)
  Change : Sum  AccumDataTypeStr=fixdt(1,4,0)  OutDataTypeStr=fixdt(1,4,0)
  Change1 : Delay  DelayLength=1
  Save_Direction : Switch  Criteria=u2 ~= 0  Threshold=0.1  OutDataTypeStr=Inherit: Inherit via back propagation
  Scope6 : Scope  NumInputPorts=4
  T_count_switch : Switch  Threshold=1  OutDataTypeStr=Inherit: Inherit via back propagation
  TrnLeft : Sum  Inputs=+-  AccumDataTypeStr=fixdt(1,4,0)  OutDataTypeStr=fixdt(1,4,0)
  TrnRight : Sum  Inputs=+-  AccumDataTypeStr=fixdt(1,4,0)  OutDataTypeStr=fixdt(1,4,0)
  TurnLeft : Constant  Value=-1  OutDataTypeStr=fixdt(1,4,0)  SampleTime=-1
  TurnRight : Constant  OutDataTypeStr=fixdt(1,4,0)  SampleTime=-1
  count_old : Delay  DelayLength=1
  count_old1 : Delay  DelayLength=1
  count_old2 : Delay  DelayLength=1
  count_old_switch : Switch  Criteria=u2 ~= 0  OutDataTypeStr=Inherit: Inherit via back propagation
  count_old_switch1 : Switch  Criteria=u2 ~= 0  OutDataTypeStr=Inherit: Inherit via back propagation
  new_value : Delay  DelayLength=1
  nothing : Constant  Value=0  OutDataTypeStr=fixdt(1,4,0)  SampleTime=-1
  nothing1 : Constant  Value=0  OutDataTypeStr=fixdt(1,4,0)  SampleTime=-1
  speed_old_switch : Switch  Threshold=1  OutDataTypeStr=Inherit: Inherit via back propagation
  Dir : Outport
  wires:
  A/1 -> TrnLeft/2, Add/1, count_old_switch/1
  count_old_switch/1 -> count_old/1
  count_old/1 -> count_old_switch/3, Add/2
  TurnRight/1 -> T_count_switch/1
  Add/1 -> TrnRight/1, count_old_switch/2
  T_count_switch/1 -> Change/1, Add2/1
  Save_Direction/1 -> count_old2/1
  B/1 -> TrnRight/2, Add1/1, count_old_switch1/1
  count_old_switch1/1 -> count_old1/1
  count_old1/1 -> count_old_switch1/3, Add1/2
  Add1/1 -> TrnLeft/1, count_old_switch1/2
  TrnRight/1 -> Scope6/1, T_count_switch/2
  new_value/1 -> Save_Direction/1
  TrnLeft/1 -> speed_old_switch/2, Scope6/2
  TurnLeft/1 -> speed_old_switch/1
  nothing/1 -> speed_old_switch/3
  nothing1/1 -> T_count_switch/3
  speed_old_switch/1 -> Change/2, Add2/2
  Add2/1 -> Scope6/4, new_value/1
  Change/1 -> Change1/1
  Change1/1 -> Scope6/3, Save_Direction/2
  count_old2/1 -> Save_Direction/3, Dir/1

== system gm_Encoder_Zynq_vnl/IncreEncoder_V19/Counter_speed ==
  note: 1 for one cycle if edge recognized
  note: Check if count is to small
  note: Check if count is to big
  note: Reset
  note: Count
  Enable_ctr : Inport
  Reset : Inport  Port=2
  IncsPerTurn : Inport  Port=3
  Add1 : Sum  AccumDataTypeStr=int16  OutDataTypeStr=uint16
  Constant1 : Constant  Value=0  OutDataTypeStr=uint16  SampleTime=-1
  Constant2 : Constant  OutDataTypeStr=int8  SampleTime=-1
  Constant3 : Constant  Value=0  OutDataTypeStr=int8  SampleTime=-1
  Constant4 : Constant  Value=10  OutDataTypeStr=uint16  SampleTime=-1
  Detec_edge : Sum  Inputs=+-  AccumDataTypeStr=int8  OutDataTypeStr=int8
  Relational Operator : RelationalOperator  OutDataTypeStr=boolean  RndMeth=Nearest
  Reset_flag : Sum  Inputs=+-  AccumDataTypeStr=uint8  OutDataTypeStr=uint8
  Reset_when_overflow : Sum
  Resett_switch1 : Switch  Criteria=u2 ~= 0
  Resett_switch2 : Switch  Criteria=u2 ~= 0
  reset_old{,1..3} (4 alike) : Delay  DelayLength=1
  reset_old_switch : Switch  Criteria=u2 ~= 0
  reset_old_switch1 : Switch  Criteria=u2 ~= 0
  speed_old_switch1 : Switch  Threshold=1
  count : Outport
  wires:
  Reset/1 -> Reset_flag/1, reset_old_switch/1
  reset_old_switch/1 -> reset_old/1
  reset_old/1 -> reset_old_switch/3, Reset_flag/2
  Reset_flag/1 -> reset_old_switch/2, Resett_switch2/2
  Enable_ctr/1 -> Detec_edge/1, reset_old_switch1/1
  reset_old_switch1/1 -> reset_old1/1
  reset_old1/1 -> reset_old_switch1/3, Detec_edge/2
  Detec_edge/1 -> speed_old_switch1/2, reset_old_switch1/2  "1 for one cycle if edge recognized"
  Add1/1 -> Resett_switch2/3
  reset_old2/1 -> Relational Operator/1, Add1/2, count/1
  speed_old_switch1/1 -> Add1/1
  Constant3/1 -> speed_old_switch1/3
  Constant2/1 -> speed_old_switch1/1
  Constant4/1 -> Reset_when_overflow/1
  Reset_when_overflow/1 -> reset_old3/1
  Resett_switch1/1 -> reset_old2/1
  Relational Operator/1 -> Resett_switch1/2
  Constant1/1 -> Resett_switch2/1, Resett_switch1/1
  IncsPerTurn/1 -> Reset_when_overflow/2
  Resett_switch2/1 -> Resett_switch1/3
  reset_old3/1 -> Relational Operator/2

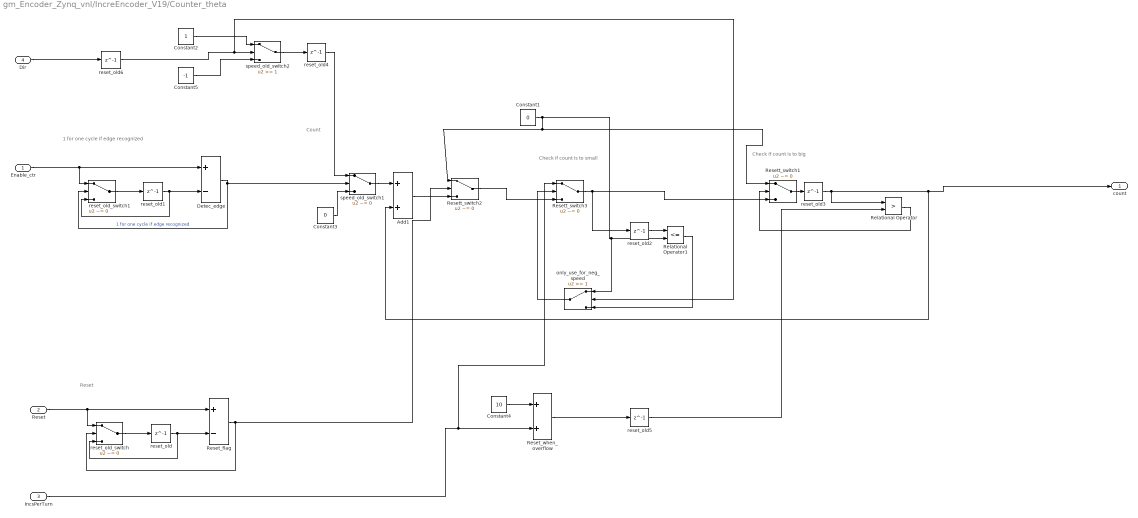
== system gm_Encoder_Zynq_vnl/IncreEncoder_V19/Counter_theta ==
  note: 1 for one cycle if edge recognized
  note: Reset
  note: Count
  note: Check if count is to big
  note: Check if count is to small
  Enable_ctr : Inport
  Reset : Inport  Port=2
  IncsPerTurn : Inport  Port=3
  Dir : Inport  Port=4
  Add1 : Sum  AccumDataTypeStr=int16  OutDataTypeStr=int16
  Constant1 : Constant  Value=0  OutDataTypeStr=int16  SampleTime=-1
  Constant2 : Constant  OutDataTypeStr=int16  SampleTime=-1
  Constant3 : Constant  Value=0  OutDataTypeStr=int16  SampleTime=-1
  Constant4 : Constant  Value=10  OutDataTypeStr=int16  SampleTime=-1
  Constant5 : Constant  Value=-1  OutDataTypeStr=int16  SampleTime=-1
  Detec_edge : Sum  Inputs=+-  AccumDataTypeStr=int8  OutDataTypeStr=int8
  Relational Operator : RelationalOperator  Operator=>  OutDataTypeStr=boolean  RndMeth=Nearest
  Relational Operator1 : RelationalOperator  Operator=<=  OutDataTypeStr=boolean  RndMeth=Nearest
  Reset_flag : Sum  Inputs=+-  AccumDataTypeStr=uint8  OutDataTypeStr=uint8
  Reset_when_overflow : Sum  OutDataTypeStr=int16
  Resett_switch1 : Switch  Criteria=u2 ~= 0  OutDataTypeStr=int16
  Resett_switch2 : Switch  Criteria=u2 ~= 0  OutDataTypeStr=int16
  Resett_switch3 : Switch  Criteria=u2 ~= 0  OutDataTypeStr=int16
  only_use_for_neg_speed : Switch  Threshold=1
  reset_old{,1..6} (7 alike) : Delay  DelayLength=1
  reset_old_switch : Switch  Criteria=u2 ~= 0
  reset_old_switch1 : Switch  Criteria=u2 ~= 0
  speed_old_switch1 : Switch  Criteria=u2 ~= 0
  speed_old_switch2 : Switch  Threshold=1
  count : Outport
  wires:
  Reset/1 -> Reset_flag/1, reset_old_switch/1
  reset_old_switch/1 -> reset_old/1
  reset_old/1 -> reset_old_switch/3, Reset_flag/2
  Reset_flag/1 -> reset_old_switch/2, Resett_switch2/2
  Enable_ctr/1 -> Detec_edge/1, reset_old_switch1/1
  reset_old_switch1/1 -> reset_old1/1
  reset_old1/1 -> reset_old_switch1/3, Detec_edge/2
  Detec_edge/1 -> speed_old_switch1/2, reset_old_switch1/2  "1 for one cycle if edge recognized"
  Add1/1 -> Resett_switch2/3
  speed_old_switch1/1 -> Add1/1
  Constant3/1 -> speed_old_switch1/3
  Constant2/1 -> speed_old_switch2/1
  Constant4/1 -> Reset_when_overflow/1
  Reset_when_overflow/1 -> reset_old5/1
  IncsPerTurn/1 -> Resett_switch3/1, Reset_when_overflow/2
  Dir/1 -> reset_old6/1
  Constant5/1 -> speed_old_switch2/3
  speed_old_switch2/1 -> reset_old4/1
  reset_old3/1 -> Add1/2, count/1, Relational Operator/1
  Resett_switch1/1 -> reset_old3/1
  Relational Operator/1 -> Resett_switch1/2
  Constant1/1 -> Resett_switch2/1, Resett_switch1/1, only_use_for_neg_speed/1, Relational Operator1/2
  Resett_switch3/1 -> reset_old2/1, Resett_switch1/3
  Resett_switch2/1 -> Resett_switch3/3
  reset_old2/1 -> Relational Operator1/1
  Relational Operator1/1 -> only_use_for_neg_speed/3
  only_use_for_neg_speed/1 -> Resett_switch3/2
  reset_old4/1 -> speed_old_switch1/1
  reset_old5/1 -> Relational Operator/2
  reset_old6/1 -> only_use_for_neg_speed/2, speed_old_switch2/2

== system gm_Encoder_Zynq_vnl/IncreEncoder_V19/Counter_theta_ele ==
  note: 1 for one cycle if edge recognized
  note: Reset
  note: Count
  note: Check if count is to big
  note: Check if count is to small
  Enable_ctr : Inport
  Reset : Inport  Port=2
  IncsPerTurn : Inport  Port=3
  Dir : Inport  Port=4
  Add1 : Sum  AccumDataTypeStr=int16  OutDataTypeStr=int16
  Constant1 : Constant  Value=0  OutDataTypeStr=int16  SampleTime=-1
  Constant2 : Constant  OutDataTypeStr=int16  SampleTime=-1
  Constant3 : Constant  Value=0  OutDataTypeStr=int16  SampleTime=-1
  Constant5 : Constant  Value=-1  OutDataTypeStr=int16  SampleTime=-1
  Detec_edge : Sum  Inputs=+-  AccumDataTypeStr=int8  OutDataTypeStr=int8
  Relational Operator : RelationalOperator  Operator=>  OutDataTypeStr=boolean  RndMeth=Nearest
  Relational Operator1 : RelationalOperator  Operator=<=  OutDataTypeStr=boolean  RndMeth=Nearest
  Reset_flag : Sum  Inputs=+-  AccumDataTypeStr=uint8  OutDataTypeStr=uint8
  Resett_switch1 : Switch  Criteria=u2 ~= 0  OutDataTypeStr=int16
  Resett_switch2 : Switch  Criteria=u2 ~= 0  OutDataTypeStr=int16
  Resett_switch3 : Switch  Criteria=u2 ~= 0  OutDataTypeStr=int16
  only_use_for_neg_speed : Switch  Threshold=1
  reset_old{,1..5} (6 alike) : Delay  DelayLength=1
  reset_old_switch : Switch  Criteria=u2 ~= 0
  reset_old_switch1 : Switch  Criteria=u2 ~= 0
  speed_old_switch1 : Switch  Criteria=u2 ~= 0
  speed_old_switch2 : Switch  Threshold=1
  count : Outport
  wires:
  Reset/1 -> Reset_flag/1, reset_old_switch/1
  reset_old_switch/1 -> reset_old/1
  reset_old/1 -> reset_old_switch/3, Reset_flag/2
  Reset_flag/1 -> reset_old_switch/2, Resett_switch2/2
  Enable_ctr/1 -> Detec_edge/1, reset_old_switch1/1
  reset_old_switch1/1 -> reset_old1/1
  reset_old1/1 -> reset_old_switch1/3, Detec_edge/2
  Detec_edge/1 -> speed_old_switch1/2, reset_old_switch1/2  "1 for one cycle if edge recognized"
  Add1/1 -> Resett_switch2/3
  speed_old_switch1/1 -> Add1/1
  Constant3/1 -> speed_old_switch1/3
  Constant2/1 -> speed_old_switch2/1
  IncsPerTurn/1 -> Resett_switch3/1, Relational Operator/2
  Dir/1 -> reset_old5/1
  Constant5/1 -> speed_old_switch2/3
  speed_old_switch2/1 -> reset_old4/1
  reset_old3/1 -> Add1/2, count/1, Relational Operator/1
  Resett_switch1/1 -> reset_old3/1
  Relational Operator/1 -> Resett_switch1/2
  Constant1/1 -> Resett_switch2/1, only_use_for_neg_speed/1, Relational Operator1/2, Resett_switch1/1
  Resett_switch3/1 -> reset_old2/1, Resett_switch1/3
  Resett_switch2/1 -> Resett_switch3/3
  reset_old2/1 -> Relational Operator1/1
  Relational Operator1/1 -> only_use_for_neg_speed/3
  only_use_for_neg_speed/1 -> Resett_switch3/2
  reset_old4/1 -> speed_old_switch1/1
  reset_old5/1 -> speed_old_switch2/2, only_use_for_neg_speed/2

== system gm_Encoder_Zynq_vnl/IncreEncoder_V19/n_aus_theta ==
  note: Detect each edge of the encoder
  count : Inport
  T : Inport  Port=2
  ProtectThetaLimit : Inport  Port=3
  Add : Sum  Inputs=+-
  Add1 : Sum
  Constant : Constant  Value=0  OutDataTypeStr=fixdt(0,30,24)  SampleTime=-1
  Constant1 : Constant  Value=0  OutDataTypeStr=fixdt(0,30,24)  SampleTime=-1
  Constant2 : Constant  Value=0  OutDataTypeStr=fixdt(0,30,24)  SampleTime=-1
  Logical Operator : Logic  AllPortsSameDT=off  OutDataTypeStr=boolean
  ProtectOverflow_T_count : Switch  Threshold=50
  ProtectOverflow_rps : Switch  Threshold=50  OutDataTypeStr=fixdt(0,30,24)
  ProtectToUseOmegaIfThetaJump : RelationalOperator  OutDataTypeStr=boolean  RndMeth=Nearest
  T_count : Delay  DelayLength=1
  T_count_switch : Switch  Criteria=u2 ~= 0
  count_old : Delay  DelayLength=1
  count_old_switch : Switch  Criteria=u2 ~= 0
  speed_old : Delay  DelayLength=1
  speed_old_switch : Switch  Criteria=u2 ~= 0
  rps : Outport
  wires:
  count_old_switch/1 -> count_old/1
  count_old/1 -> count_old_switch/3, Add/2
  Constant/1 -> T_count_switch/1
  Add/1 -> count_old_switch/2, Logical Operator/1, T_count_switch/2
  Constant1/1 -> ProtectOverflow_T_count/1
  ProtectOverflow_rps/1 -> rps/1
  Constant2/1 -> ProtectOverflow_rps/1
  speed_old_switch/1 -> ProtectOverflow_rps/3, speed_old/1
  speed_old/1 -> speed_old_switch/3
  T/1 -> Add1/1
  ProtectOverflow_T_count/1 -> T_count/1
  T_count/1 -> Add1/2
  Add1/1 -> speed_old_switch/1, T_count_switch/3
  count/1 -> ProtectToUseOmegaIfThetaJump/1, Add/1, count_old_switch/1
  T_count_switch/1 -> ProtectOverflow_rps/2, ProtectOverflow_T_count/2, ProtectOverflow_T_count/3
  ProtectToUseOmegaIfThetaJump/1 -> Logical Operator/2
  Logical Operator/1 -> speed_old_switch/2
  ProtectThetaLimit/1 -> ProtectToUseOmegaIfThetaJump/2

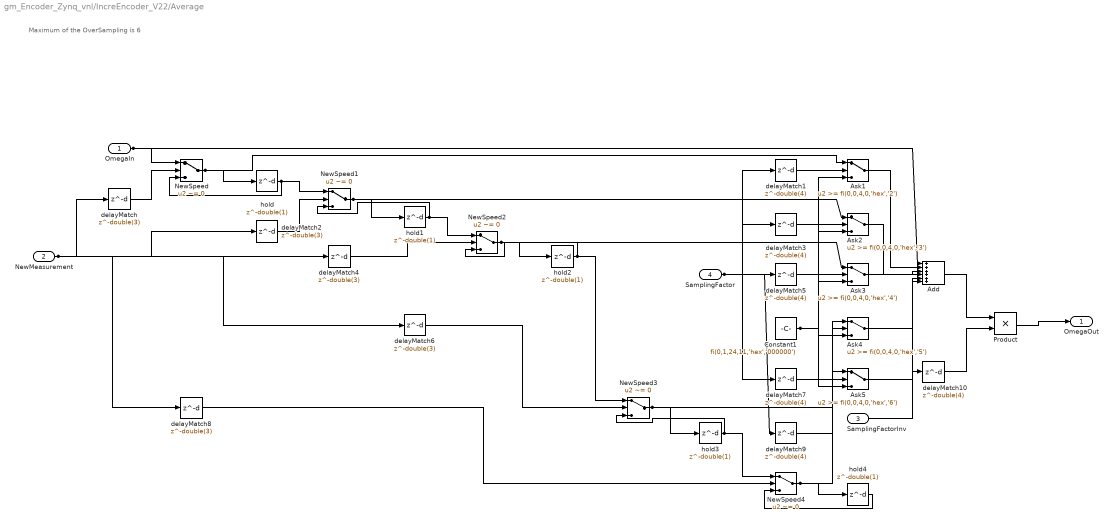
== system gm_Encoder_Zynq_vnl/IncreEncoder_V22/Average ==
  note: Maximum of the OverSampling is 6
  "OmegaIn " : Inport  PortDimensions=1  SampleTime=2e-08
  NewMeasurement : Inport  Port=2  PortDimensions=1  SampleTime=2e-08
  SamplingFactorInv : Inport  Port=3  PortDimensions=1  SampleTime=2e-08
  SamplingFactor : Inport  Port=4  PortDimensions=1  SampleTime=2e-08
  Add : Sum  Inputs=++++++  AccumDataTypeStr=fixdt(1, 24, 11)  OutDataTypeStr=fixdt(1, 24, 11)  SampleTime=2e-08
  Ask1 : Switch  Threshold=fi(0,0,4,0,'hex','2')  OutDataTypeStr=fixdt(1, 24, 11)  SampleTime=2e-08
  Ask2 : Switch  Threshold=fi(0,0,4,0,'hex','3')  OutDataTypeStr=fixdt(1, 24, 11)  SampleTime=2e-08
  Ask3 : Switch  Threshold=fi(0,0,4,0,'hex','4')  OutDataTypeStr=fixdt(1, 24, 11)  SampleTime=2e-08
  Ask4 : Switch  Threshold=fi(0,0,4,0,'hex','5')  OutDataTypeStr=fixdt(1, 24, 11)  SampleTime=2e-08
  Ask5 : Switch  Threshold=fi(0,0,4,0,'hex','6')  OutDataTypeStr=fixdt(1, 24, 11)  SampleTime=2e-08
  Constant1 : Constant  Value=fi(0,1,24,11,'hex','000000')  OutDataTypeStr=fixdt(1, 24, 11)  SampleTime=-1
  NewSpeed{,1..4} (5 alike) : Switch  Criteria=u2 ~= 0  Threshold=double(0)  OutDataTypeStr=fixdt(1, 24, 11)  SampleTime=2e-08
  Product : Product  Inputs=**  OutDataTypeStr=fixdt(1, 24, 11)  SampleTime=2e-08
  delayMatch{,2,4,6,8} (5 alike) : Delay  DelayLength=double(3)  InitialCondition=0  InputProcessing=Inherited  SampleTime=2e-08
  delayMatch{1,3,5,7,9..10} (6 alike) : Delay  DelayLength=double(4)  InitialCondition=0  InputProcessing=Inherited  SampleTime=2e-08
  hold{,1..4} (5 alike) : Delay  DelayLength=double(1)  InitialCondition=0  InputProcessing=Inherited  SampleTime=2e-08
  OmegaOut : Outport
  wires:
  hold4/1 -> NewSpeed4/3
  SamplingFactor/1 -> delayMatch1/1, delayMatch3/1, delayMatch5/1, delayMatch7/1, delayMatch9/1
  SamplingFactorInv/1 -> delayMatch10/1
  NewMeasurement/1 -> delayMatch/1, delayMatch2/1, delayMatch4/1, delayMatch6/1, delayMatch8/1
  "OmegaIn "/1 -> NewSpeed/1, Add/1
  NewSpeed4/1 -> hold4/1, Ask5/1
  NewSpeed3/1 -> hold3/1, Ask4/1
  hold3/1 -> NewSpeed4/1, NewSpeed3/3
  NewSpeed2/1 -> hold2/1, Ask3/1
  hold2/1 -> NewSpeed3/1, NewSpeed2/3
  NewSpeed1/1 -> hold1/1, Ask2/1
  hold1/1 -> NewSpeed2/1, NewSpeed1/3
  NewSpeed/1 -> hold/1, Ask1/1
  hold/1 -> NewSpeed1/1, NewSpeed/3
  delayMatch9/1 -> Ask5/2
  delayMatch8/1 -> NewSpeed4/2
  delayMatch7/1 -> Ask4/2
  delayMatch6/1 -> NewSpeed3/2
  delayMatch5/1 -> Ask3/2
  delayMatch4/1 -> NewSpeed2/2
  delayMatch3/1 -> Ask2/2
  delayMatch2/1 -> NewSpeed1/2
  Product/1 -> OmegaOut/1
  Constant1/1 -> Ask1/3, Ask2/3, Ask3/3, Ask4/3, Ask5/3
  Ask5/1 -> Add/6
  Ask4/1 -> Add/5
  Ask3/1 -> Add/4
  Ask2/1 -> Add/3
  Ask1/1 -> Add/2
  Add/1 -> Product/1
  delayMatch1/1 -> Ask1/2
  delayMatch10/1 -> Product/2
  delayMatch/1 -> NewSpeed/2
